simulink model "sampleModel1961"  (R2023a)
settings: Solver=VariableStepAuto  StartTime=0.0  StopTime=10.0  RelTol=1e-3
libraries: hdlsllib x8, simulink x3
settings Model: Creator=user1  LastModifiedBy=user1

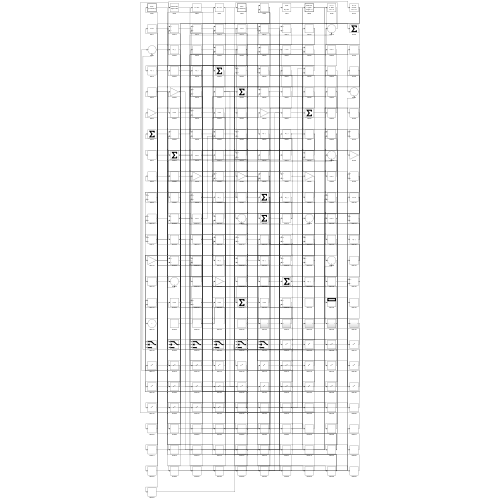
[thumbnail: Simulink's stored preview of the top-level diagram]
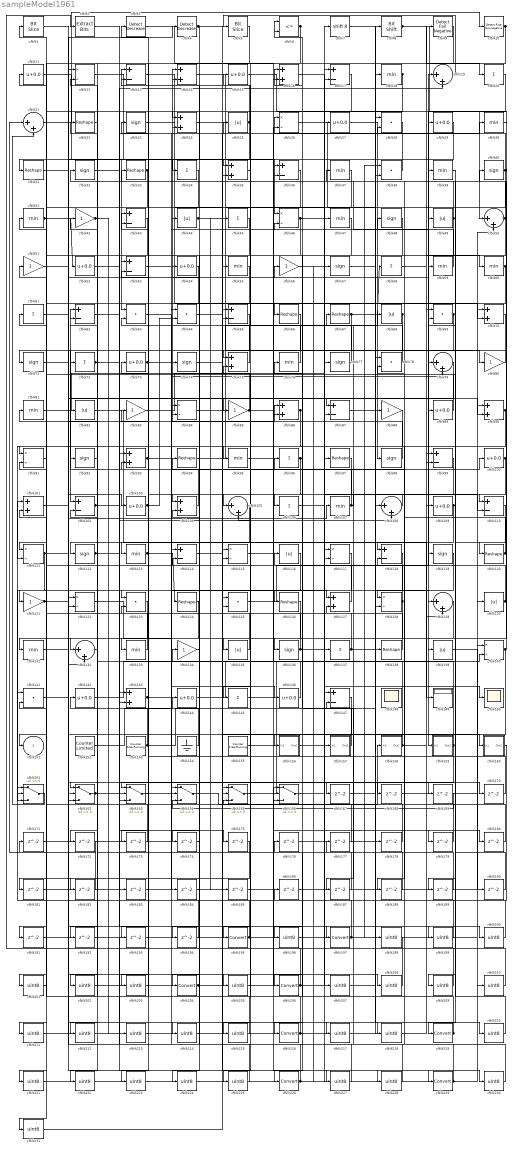
== system sampleModel1961 ==
  cfblk1 : hdlsllib/Logic and Bit Operations/Bit Slice  lidx=7  ridx=0
  cfblk10 : hdlsllib/Logic and Bit Operations/Detect Rise Nonnegative  vinit=0  OutDataTypeStr=boolean
  cfblk{11,15,27,29,52,54,73,89,100,103,109,142,144,146} (14 alike) : Bias  Bias=0.0  SaturateOnIntegerOverflow=off
  cfblk{14,16,24,35,70,75,86,90,93,101,104,127,143} (13 alike) : Sum
  cfblk{13,17,36,43,53,62,65,87,99,102,110,114,118,147} (14 alike) : Sum  Inputs=+-
  cfblk{19,21,50,79,105,108,129,132} (8 alike) : Sum  Inputs=|++
  cfblk{20,34,45,58,61,72,96,106,137,145} (10 alike) : Sum  Inputs=+
  cfblk{18,30,37,39,41,47,55,59..60,76,81,95,107,113,131,133} (16 alike) : MinMax
  cfblk{12,26,46,84,91,111,115,117,122,128,140} (11 alike) : Product  Inputs=*/  RndMeth=Zero  SaturateOnIntegerOverflow=on
  cfblk{23,32,40,48,57,71,74,77,92,98,112,119,136} (13 alike) : Signum
  cfblk{25,44,49,68,82,116,130,135,139} (9 alike) : Abs  SaturateOnIntegerOverflow=off
  cfblk{22,31,33,66..67,94,97,120,124,126,138} (11 alike) : Reshape
  cfblk{42,51,56,80,83,85,88,121,134} (9 alike) : Gain
  cfblk{28,38,63..64,69,78,123,125,141} (9 alike) : DotProduct  OutDataTypeStr=Inherit: Inherit via internal rule
  cfblk148 : Scope
      settings: Floating=on
  cfblk149 : Display
  cfblk150 : Scope
  cfblk152 : hdlsllib/Sources/Counter Limited  uplimit=7  tsamp=-1
  cfblk153 : hdlsllib/Sources/Counter Free-Running  NumBits=16  tsamp=-1
  cfblk154 : Ground
  cfblk155 : hdlsllib/Sources/Counter Free-Running  NumBits=16  tsamp=-1
  cfblk156 : Subsystem
      settings: LibrarySourceBlock=|
      | hdlsllib/Ports &
      | Subsystems/Subsystem
  cfblk157 : Subsystem
      settings: LibrarySourceBlock=|
      | hdlsllib/Ports &
      | Subsystems/Subsystem
  cfblk158 : Subsystem
      settings: LibrarySourceBlock=|
      | hdlsllib/Ports &
      | Subsystems/Subsystem
  cfblk159 : Subsystem
      settings: LibrarySourceBlock=|
      | hdlsllib/Ports &
      | Subsystems/Subsystem
  cfblk160 : Subsystem
      settings: LibrarySourceBlock=|
      | hdlsllib/Ports &
      | Subsystems/Subsystem
  cfblk{161..166} (6 alike) : Switch  SaturateOnIntegerOverflow=off  InputSameDT=off
  cfblk{167..194} (28 alike) : Delay  SampleTime=1
  cfblk{195,197,204,206,216,219,226,229} (8 alike) : DataTypeConversion  SaturateOnIntegerOverflow=off  RndMeth=Floor
  cfblk{196,198..203,205,207..215,217..218,220..225,227..228,230..231} (29 alike) : DataTypeConversion  OutDataTypeStr=uint8  SaturateOnIntegerOverflow=off  RndMeth=Floor
  cfblk2 : simulink/Logic and Bit Operations/Extract Bits  bitsToExtract=Upper half  numBits=8  bitIdxRange=[0 7]  outScalingMode=Preserve fixed-point scaling
      settings: LibrarySourceBlock=|
      | hdlsllib/Logic and Bit
      | Operations/Extract Bits
  cfblk3 : simulink/Logic and Bit Operations/Detect Decrease  vinit=0.0  OutDataTypeStr=boolean
      settings: LibrarySourceBlock=|
      | hdlsllib/Logic and Bit
      | Operations/Detect
      | Decrease
  cfblk4 : simulink/Logic and Bit Operations/Detect Decrease  vinit=0.0  OutDataTypeStr=boolean
      settings: LibrarySourceBlock=|
      | hdlsllib/Logic and Bit
      | Operations/Detect
      | Decrease
  cfblk5 : hdlsllib/Logic and Bit Operations/Bit Slice  lidx=7  ridx=0
  cfblk6 : RelationalOperator  Operator=<=  OutDataTypeStr=boolean  InputSameDT=off
  cfblk7 : ArithShift  BitShiftNumber=8
  cfblk8 : hdlsllib/Logic and Bit Operations/Bit Shift  mode=Shift Left Logical  N=0
  cfblk9 : hdlsllib/Logic and Bit Operations/Detect Fall Negative  vinit=0  OutDataTypeStr=boolean
  cfblk151 : Outport  VectorParamsAs1DForOutWhenUnconnected=off
  wires:
  cfblk111/1 -> cfblk161/3, cfblk107/1, cfblk205/1
  cfblk29/1 -> cfblk63/1
  cfblk34/1 -> cfblk113/1
  cfblk8/1 -> cfblk136/1, cfblk20/1
  cfblk13/1 -> cfblk66/1
  cfblk88/1 -> cfblk206/1
  cfblk104/1 -> cfblk13/1
  cfblk128/1 -> cfblk116/1, cfblk163/1
  cfblk120/1 -> cfblk32/1, cfblk96/1
  cfblk125/1 -> cfblk19/1
  cfblk24/1 -> cfblk80/1
  cfblk40/1 -> cfblk26/1, cfblk65/2, cfblk163/3
  cfblk50/1 -> cfblk159/1(In1), cfblk16/1
  cfblk19/1 -> cfblk5/1
  cfblk78/1 -> cfblk14/1
  cfblk37/1 -> cfblk133/1
  cfblk20/1 -> cfblk119/1
  cfblk21/1 -> cfblk10/1
  cfblk14/1 -> cfblk157/1(In1)
  cfblk69/1 -> cfblk102/1, cfblk212/1
  cfblk77/1 -> cfblk63/2
  cfblk76/1 -> cfblk15/1
  cfblk92/1 -> cfblk112/1
  cfblk137/1 -> cfblk127/2, cfblk220/1
  cfblk113/1 -> cfblk124/1, cfblk146/1
  cfblk98/1 -> cfblk44/1
  cfblk155/1 -> cfblk109/1
  cfblk75/1 -> cfblk33/1
  cfblk27/1 -> cfblk98/1
  cfblk12/1 -> cfblk55/1
  cfblk152/1 -> cfblk144/1
  cfblk90/1 -> cfblk128/1, cfblk111/2
  cfblk142/1 -> cfblk47/1
  cfblk146/1 -> cfblk23/1
  cfblk163/1 -> cfblk100/1
  cfblk108/1 -> cfblk106/1
  cfblk138/1 -> cfblk51/1
  cfblk49/1 -> cfblk104/1, cfblk6/2, cfblk209/1
  cfblk5/1 -> cfblk131/1
  cfblk60/1 -> cfblk120/1, cfblk95/1
  cfblk11/1 -> cfblk46/1
  cfblk165/1 -> cfblk8/1
  cfblk67/1 -> cfblk58/1, cfblk87/2
  cfblk107/1 -> cfblk62/1, cfblk67/1
  cfblk126/1 -> cfblk135/1
  cfblk102/1 -> cfblk24/2, cfblk167/1
  cfblk95/1 -> cfblk36/1
  cfblk156/1(Out1) -> cfblk68/1
  cfblk144/1 -> cfblk26/2
  cfblk103/1 -> cfblk43/1, cfblk64/2
  cfblk26/1 -> cfblk138/1
  cfblk32/1 -> cfblk87/1
  cfblk85/1 -> cfblk74/1, cfblk180/1, cfblk217/1
  cfblk23/1 -> cfblk65/1
  cfblk100/1 -> cfblk118/1, cfblk187/1, cfblk188/1
  cfblk97/1 -> cfblk204/1
  cfblk59/1 -> cfblk37/1
  cfblk86/1 -> cfblk151/1, cfblk145/1
  cfblk82/1 -> cfblk149/1
  cfblk96/1 -> cfblk156/1(In1), cfblk193/1, cfblk194/1
  cfblk154/1 -> cfblk142/1
  cfblk135/1 -> cfblk54/1
  cfblk116/1 -> cfblk161/2
  cfblk115/1 -> cfblk229/1
  cfblk25/1 -> cfblk53/1, cfblk13/2, cfblk71/1
  cfblk57/1 -> cfblk49/1
  cfblk4/1 -> cfblk70/2, cfblk34/1
  cfblk73/1 -> cfblk59/1, cfblk79/2
  cfblk15/1 -> cfblk50/1
  cfblk55/1 -> cfblk72/1
  cfblk9/1 -> cfblk195/1
  cfblk6/1 -> cfblk92/1, cfblk16/2
  cfblk47/1 -> cfblk126/1
  cfblk109/1 -> cfblk132/1, cfblk79/1
  cfblk131/1 -> cfblk56/1
  cfblk122/1 -> cfblk164/2
  cfblk79/1 -> cfblk122/2
  cfblk65/1 -> cfblk123/1
  cfblk41/1 -> cfblk52/1, cfblk218/1
  cfblk133/1 -> cfblk11/1
  cfblk10/1 -> cfblk166/3, cfblk172/1, cfblk173/1
  cfblk31/1 -> cfblk35/1
  cfblk3/1 -> cfblk36/2
  cfblk1/1 -> cfblk132/2
  cfblk30/1 -> cfblk110/1
  cfblk53/1 -> cfblk46/2
  cfblk121/1 -> cfblk4/1, cfblk86/2
  cfblk81/1 -> cfblk64/1
  cfblk114/1 -> cfblk160/1(In1)
  cfblk46/1 -> cfblk165/2, cfblk110/2
  cfblk140/1 -> cfblk40/1, cfblk162/3
  cfblk112/1 -> cfblk175/1, cfblk213/1
  cfblk143/1 -> cfblk140/2, cfblk48/1
  cfblk68/1 -> cfblk121/1, cfblk223/1
  cfblk132/1 -> cfblk82/1
  cfblk147/1 -> cfblk226/1
  cfblk44/1 -> cfblk28/2, cfblk127/1, cfblk185/1
  cfblk94/1 -> cfblk27/1
  cfblk7/1 -> cfblk90/2
  cfblk2/1 -> cfblk197/1
  cfblk83/1 -> cfblk7/1
  cfblk159/1(Out1) -> cfblk81/1, cfblk162/2
  cfblk16/1 -> cfblk150/1
  cfblk164/1 -> cfblk158/1(In1)
  cfblk72/1 -> cfblk108/2, cfblk29/1
  cfblk71/1 -> cfblk89/1
  cfblk153/1 -> cfblk18/1, cfblk78/1, cfblk102/2
  cfblk42/1 -> cfblk22/1, cfblk183/1
  cfblk33/1 -> cfblk143/2, cfblk162/1
  cfblk89/1 -> cfblk1/1
  cfblk18/1 -> cfblk24/1, cfblk105/1
  cfblk87/1 -> cfblk129/1
  cfblk93/1 -> cfblk25/1, cfblk125/2
  cfblk52/1 -> cfblk19/2
  cfblk127/1 -> cfblk86/1
  cfblk38/1 -> cfblk31/1
  cfblk43/1 -> cfblk91/1
  cfblk51/1 -> cfblk103/1
  cfblk162/1 -> cfblk12/2, cfblk170/1
  cfblk130/1 -> cfblk6/1, cfblk41/1
  cfblk28/1 -> cfblk85/1
  cfblk80/1 -> cfblk75/1
  cfblk56/1 -> cfblk137/1
  cfblk99/1 -> cfblk216/1
  cfblk58/1 -> cfblk60/1
  cfblk136/1 -> cfblk14/2, cfblk118/2
  cfblk39/1 -> cfblk219/1
  cfblk161/1 -> cfblk21/2
  cfblk158/1(Out1) -> cfblk129/2, cfblk93/2
  cfblk74/1 -> cfblk125/1
  cfblk157/1(Out1) -> cfblk76/1
  cfblk62/1 -> cfblk30/1
  cfblk54/1 -> cfblk111/1
  cfblk70/1 -> cfblk139/1
  cfblk129/1 -> cfblk168/1
  cfblk168/1 -> cfblk140/1
  cfblk64/1 -> cfblk169/1
  cfblk169/1 -> cfblk164/3
  cfblk170/1 -> cfblk53/2
  cfblk171/1 -> cfblk164/1
  cfblk172/1 -> cfblk21/1
  cfblk173/1 -> cfblk93/1
  cfblk66/1 -> cfblk174/1
  cfblk174/1 -> cfblk104/2
  cfblk176/1 -> cfblk38/2
  cfblk177/1 -> cfblk12/1
  cfblk178/1 -> cfblk141/2
  cfblk145/1 -> cfblk179/1
  cfblk179/1 -> cfblk165/1
  cfblk180/1 -> cfblk165/3
  cfblk36/1 -> cfblk181/1
  cfblk181/1 -> cfblk90/1
  cfblk22/1 -> cfblk182/1
  cfblk182/1 -> cfblk161/1
  cfblk183/1 -> cfblk35/2
  cfblk63/1 -> cfblk184/1
  cfblk185/1 -> cfblk166/2
  cfblk160/1(Out1) -> cfblk186/1
  cfblk186/1 -> cfblk128/2
  cfblk187/1 -> cfblk143/1
  cfblk188/1 -> cfblk75/2
  cfblk110/1 -> cfblk189/1
  cfblk189/1 -> cfblk62/2
  cfblk139/1 -> cfblk190/1
  cfblk190/1 -> cfblk69/2
  cfblk124/1 -> cfblk191/1
  cfblk191/1 -> cfblk108/1
  cfblk123/1 -> cfblk192/1
  cfblk193/1 -> cfblk50/2
  cfblk194/1 -> cfblk91/2
  cfblk195/1 -> cfblk43/2, cfblk73/1
  cfblk48/1 -> cfblk196/1
  cfblk196/1 -> cfblk9/1
  cfblk197/1 -> cfblk123/2, cfblk38/1
  cfblk167/1 -> cfblk198/1
  cfblk198/1 -> cfblk2/1
  cfblk101/1 -> cfblk199/1
  cfblk199/1 -> cfblk141/1
  cfblk166/1 -> cfblk200/1
  cfblk200/1 -> cfblk101/1
  cfblk175/1 -> cfblk201/1
  cfblk201/1 -> cfblk101/2
  cfblk45/1 -> cfblk202/1
  cfblk202/1 -> cfblk178/1
  cfblk105/1 -> cfblk203/1
  cfblk203/1 -> cfblk45/1
  cfblk204/1 -> cfblk114/2, cfblk166/1
  cfblk205/1 -> cfblk97/1
  cfblk206/1 -> cfblk171/1, cfblk83/1
  cfblk106/1 -> cfblk207/1
  cfblk207/1 -> cfblk88/1
  cfblk84/1 -> cfblk208/1
  cfblk208/1 -> cfblk94/1
  cfblk209/1 -> cfblk84/1
  cfblk210/1 -> cfblk84/2
  cfblk117/1 -> cfblk211/1
  cfblk211/1 -> cfblk28/1
  cfblk212/1 -> cfblk117/1
  cfblk213/1 -> cfblk117/2
  cfblk61/1 -> cfblk214/1
  cfblk214/1 -> cfblk69/1
  cfblk35/1 -> cfblk215/1
  cfblk215/1 -> cfblk61/1
  cfblk216/1 -> cfblk77/1, cfblk42/1, cfblk3/1
  cfblk217/1 -> cfblk99/1
  cfblk218/1 -> cfblk99/2
  cfblk219/1 -> cfblk177/1, cfblk176/1, cfblk105/2
  cfblk220/1 -> cfblk39/1
  cfblk17/1 -> cfblk221/1
  cfblk221/1 -> cfblk70/1
  cfblk119/1 -> cfblk222/1
  cfblk222/1 -> cfblk17/1
  cfblk223/1 -> cfblk17/2
  cfblk134/1 -> cfblk224/1
  cfblk224/1 -> cfblk130/1
  cfblk118/1 -> cfblk225/1
  cfblk225/1 -> cfblk134/1
  cfblk226/1 -> cfblk210/1, cfblk114/1, cfblk57/1
  cfblk141/1 -> cfblk227/1
  cfblk227/1 -> cfblk147/1
  cfblk184/1 -> cfblk228/1
  cfblk228/1 -> cfblk147/2
  cfblk229/1 -> cfblk78/2, cfblk163/2, cfblk122/1
  cfblk192/1 -> cfblk230/1
  cfblk230/1 -> cfblk115/1
  cfblk91/1 -> cfblk231/1
  cfblk231/1 -> cfblk115/2

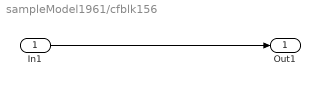
== system sampleModel1961/cfblk156 ==
  In1 : Inport
  Out1 : Outport
  wires:
  In1/1 -> Out1/1

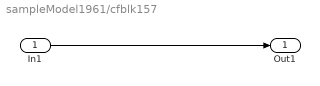
== system sampleModel1961/cfblk157 ==
  In1 : Inport
  Out1 : Outport
  wires:
  In1/1 -> Out1/1

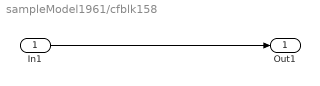
== system sampleModel1961/cfblk158 ==
  In1 : Inport
  Out1 : Outport
  wires:
  In1/1 -> Out1/1

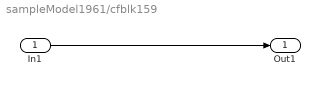
== system sampleModel1961/cfblk159 ==
  In1 : Inport
  Out1 : Outport
  wires:
  In1/1 -> Out1/1

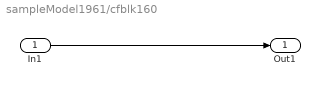
== system sampleModel1961/cfblk160 ==
  In1 : Inport
  Out1 : Outport
  wires:
  In1/1 -> Out1/1
